simulink model "dsupPeuker"  (R2014b)
settings: Solver=ode3  StartTime=0.0  StopTime=1  FixedStep=.01  RelTol=1e-3
values from neighbouring files (symbols this model uses):
  k1 = k    (= 280)    [BslipPeuker.m]
  x = xpos(end)    [BslipPeuker.m]
  x1 = xspeed(end)    [BslipPeuker.m]
  xf1 = 0    [BslipPeuker.m]
  xf2 = cos(alpha/180*pi)-xpp    [BslipPeuker.m]
  y = ypos(end)    [BslipPeuker.m]
  y1 = yspeed(end)    [BslipPeuker.m]
libraries: simulink x1
settings Model: Creator=hamidreza  LastModifiedBy=hamidreza

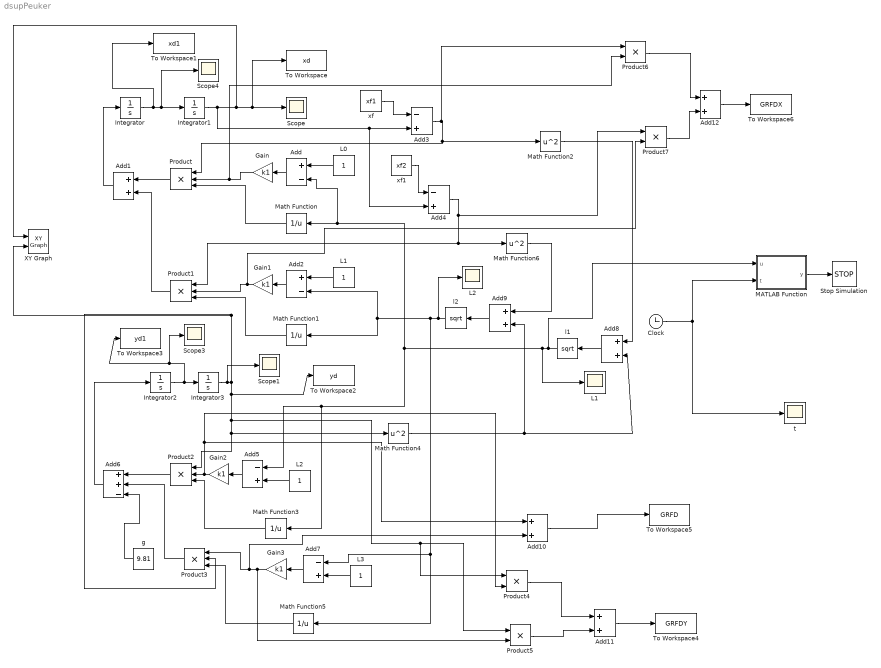
== system dsupPeuker ==
  Add : Sum  Inputs=+-
  Add{1,8..12} (6 alike) : Sum
  Add2 : Sum  Inputs=+-
  Add{3..5,7} (4 alike) : Sum  Inputs=-+
  Add6 : Sum  Inputs=++-
  Clock : Clock
  Gain{,1..3} (4 alike) : Gain  Gain=k1
  Integrator : Integrator  InitialCondition=x1
  Integrator1 : Integrator  InitialCondition=x
  Integrator2 : Integrator  InitialCondition=y1
  Integrator3 : Integrator  InitialCondition=y
  L{0..3} (4 alike) : Constant
  "L1 " : Scope
      settings: TimeRange=0.2  YMin=-0.5  YMax=2  SaveName=ScopeData2
  "L2 " : Scope
      settings: TimeRange=0.2  YMin=0.925  YMax=0.9750000000000001  SaveName=ScopeData5
  MATLAB Function : MATLAB Function  TreatAsAtomicUnit=on
  Math Function{,1,3,5} (4 alike) : Math  Operator=reciprocal  SaturateOnIntegerOverflow=on
  Math Function2 : Math  Operator=square  SaturateOnIntegerOverflow=on
  Math Function4 : Math  Operator=square  SaturateOnIntegerOverflow=on
  Math Function6 : Math  Operator=square  SaturateOnIntegerOverflow=on
  Product{,1..3} (4 alike) : Product  Inputs=3
  Product{4..7} (4 alike) : Product
  Scope{,1,3..4} (4 alike) : Scope
      Scope settings: TimeRange=0.14  YMin=0.08  YMax=0.26
      Scope1 settings: TimeRange=0.2  YMin=0.925  YMax=0.9750000000000001
      Scope3 settings: TimeRange=0.15  YMin=-0.4  YMax=0.5  SaveName=ScopeData3
      Scope4 settings: TimeRange=0.15  YMin=1.11  YMax=1.15  SaveName=ScopeData4
  Stop Simulation : Stop
  To Workspace : ToWorkspace  VariableName=xd  SaveFormat=Structure With Time  SampleTime=-1
  To Workspace1 : ToWorkspace  VariableName=xd1  SaveFormat=Structure With Time  SampleTime=-1
  To Workspace2 : ToWorkspace  VariableName=yd  SaveFormat=Structure With Time  SampleTime=-1
  To Workspace3 : ToWorkspace  VariableName=yd1  SaveFormat=Structure With Time  SampleTime=-1
  To Workspace4 : ToWorkspace  VariableName=GRFDY  SaveFormat=Structure With Time  SampleTime=-1
      settings: Save2DSignal=2-D array (concatenate along first dimension)
  To Workspace5 : ToWorkspace  VariableName=GRFD  SaveFormat=Structure With Time  SampleTime=-1
      settings: Save2DSignal=2-D array (concatenate along first dimension)
  To Workspace6 : ToWorkspace  VariableName=GRFDX  SaveFormat=Structure With Time  SampleTime=-1
      settings: Save2DSignal=2-D array (concatenate along first dimension)
  XY Graph : simulink/Sinks/XY Graph  xmin=-inf  xmax=inf  ymin=-inf  ymax=inf  st=-1
  "g " : Constant  Value=9.81
  l1 : Sqrt  SaturateOnIntegerOverflow=on
  l2 : Sqrt  SaturateOnIntegerOverflow=on
  t : Scope
      settings: TimeRange=0.2  YMin=0.925  YMax=0.9750000000000001  SaveName=ScopeData6
  xf : Constant  Value=xf1
  xf1 : Constant  Value=xf2
  wires:
  Gain/1 -> Product6/2, Product/2
  Add/1 -> Gain/1
  Math Function/1 -> Product/3
  xf/1 -> Add3/1
  Add3/1 -> Product6/1, Product/1, Math Function2/1
  L0/1 -> Add/1
  Integrator1/1 -> Add4/2, Add3/2, XY Graph/1, To Workspace/1, Scope/1
  Product/1 -> Add1/1
  Add1/1 -> Integrator/1
  Gain1/1 -> Product7/2, Product1/2
  Add2/1 -> Gain1/1
  Math Function1/1 -> Product1/3
  L1/1 -> Add2/1
  Product1/1 -> Add1/2
  xf1/1 -> Add4/1
  Add4/1 -> Product7/1, Math Function6/1, Product1/1
  Integrator2/1 -> To Workspace3/1, Scope3/1, Integrator3/1
  L2/1 -> Add5/2
  Add5/1 -> Gain2/1
  Gain2/1 -> Add10/1, Product4/2, Product2/2
  Math Function3/1 -> Product2/3
  Product2/1 -> Add6/1
  Add6/1 -> Integrator2/1
  L3/1 -> Add7/2
  Add7/1 -> Gain3/1
  Gain3/1 -> Product5/2, Add10/2, Product3/1
  Math Function5/1 -> Product3/3
  Product3/1 -> Add6/2
  Math Function2/1 -> Add8/1
  Math Function4/1 -> Add8/2, Add9/2
  Add8/1 -> l1/1
  Math Function6/1 -> Add9/1
  Add9/1 -> l2/1
  l2/1 -> Add2/2, Math Function1/1, Math Function5/1, Add7/1, "L2 "/1
  Integrator3/1 -> Scope1/1, XY Graph/2, Product3/2, Product2/1, Math Function4/1, Product5/1, Product4/1, To Workspace2/1
  "g "/1 -> Add6/3
  Clock/1 -> t/1, MATLAB Function/2(t)
  l1/1 -> MATLAB Function/1(u), Add5/1, Math Function3/1, Add/2, Math Function/1, "L1 "/1
  MATLAB Function/1(y) -> Stop Simulation/1
  Integrator/1 -> To Workspace1/1, Integrator1/1, Scope4/1
  Add10/1 -> To Workspace5/1
  Product4/1 -> Add11/1
  Product5/1 -> Add11/2
  Add11/1 -> To Workspace4/1
  Product6/1 -> Add12/1
  Product7/1 -> Add12/2
  Add12/1 -> To Workspace6/1

== matlab function dsupPeuker/MATLAB Function ==
  data: u input; y output; t input
function y = fcn(u,t)
%#codegen

if and(abs(u-1)<.005,t>.03)
    y=1;
else
    y=0;

end
